simulink model "servo_sim"  (R2023a)
settings: configuration reference "config" (kept outside this file)
model workspace (MATLAB code in the model file + MAT data in the model file):
  cmdLim = Simulink.Parameter
  cmdLim.Value = 15
  cmdLim.Description = 'Limit for controlling the maximum surface command angle.'
  cmdLim.Min = 0
  cmdLim.Max = 90
  cmdLim.DocUnits = 'deg'
  dispGain = Simulink.Parameter
  dispGain.Value = 0.75
  dispGain.Description = 'Gain applied to the displacement error.'
  dispGain.Min = 0
  dispGain.Max = []
  dispGain.DocUnits = 'deg/sec/deg'
  dispLim = Simulink.Parameter
  dispLim.Value = 30
  dispLim.Description = 'Limit for controlling the maximum commanded angle.'
  dispLim.Min = 0
  dispLim.Max = 180
  dispLim.DocUnits = 'deg'
  intGain = Simulink.Parameter
  intGain.Value = 0.5
  intGain.Description = 'Gain applied to the integral error.'
  intGain.Min = 0
  intGain.Max = []
  intGain.DocUnits = 'deg/sec/deg/sec'
  intLim = Simulink.Parameter
  intLim.Value = 5
  intLim.Description = 'Limit for controlling the maximum commanded angle.'
  intLim.Min = 0
  intLim.Max = 90
  intLim.DocUnits = 'deg'
  rateGain = Simulink.Parameter
  rateGain.Value = 2
  rateGain.Description = 'Gain applied to the rate error.'
  rateGain.Min = 0
  rateGain.Max = []
  rateGain.DocUnits = 'deg/deg/sec'
  rateLim = Simulink.Parameter
  rateLim.Value = 6
  rateLim.Description = 'Limit for controlling the maximum commanded angle.'
  rateLim.Min = 0
  rateLim.Max = 180
  rateLim.DocUnits = 'deg/sec'
  hdgGain = Simulink.Parameter
  hdgGain.Value = 0.015
  b = Simulink.Parameter
  b.Value = 0.001
  b.DataType = 'single'
  b.Complexity = 'real'
  b.Dimensions = [1 1]
  enc_line = Simulink.Parameter
  enc_line.Value = 10000
  enc_line.DataType = 'single'
  enc_line.Complexity = 'real'
  enc_line.Dimensions = [1 1]
  fc = Simulink.Parameter
  fc.Value = 0.001
  fc.DataType = 'single'
  fc.Complexity = 'real'
  fc.Dimensions = [1 1]
  flux = Simulink.Parameter
  flux.Value = 0.0125
  flux.DataType = 'single'
  flux.Complexity = 'real'
  flux.Dimensions = [1 1]
  fs = Simulink.Parameter
  fs.Value = 10000
  fs.Description = '位置环 速度环执行频率'
  fs.DataType = 'single'
  fs.Complexity = 'real'
  fs.Dimensions = [1 1]
  j = Simulink.Parameter
  j.Value = 1.9e-05
  j.DataType = 'single'
  j.Complexity = 'real'
  j.Dimensions = [1 1]
  j_inv = Simulink.Parameter
  j_inv.Value = 52631.5789474
  j_inv.DataType = 'single'
  j_inv.Complexity = 'real'
  j_inv.Dimensions = [1 1]
  kt = Simulink.Parameter
  kt.Value = 0.075
  kt.DataType = 'single'
  kt.Complexity = 'real'
  kt.Dimensions = [1 1]
  ld = Simulink.Parameter
  ld.Value = 0.00085
  ld.DataType = 'single'
  ld.Complexity = 'real'
  ld.Dimensions = [1 1]
  ld_inv = Simulink.Parameter
  ld_inv.Value = 1176.47058824
  ld_inv.DataType = 'single'
  ld_inv.Complexity = 'real'
  ld_inv.Dimensions = [1 1]
  lq = Simulink.Parameter
  lq.Value = 0.00085
  lq.DataType = 'single'
  lq.Complexity = 'real'
  lq.Dimensions = [1 1]
  lq_inv = Simulink.Parameter
  lq_inv.Value = 1176.47058824
  lq_inv.DataType = 'single'
  lq_inv.Complexity = 'real'
  lq_inv.Dimensions = [1 1]
  pn = Simulink.Parameter
  pn.Value = 4
  pn.DataType = 'single'
  pn.Complexity = 'real'
  pn.Dimensions = [1 1]
  r = Simulink.Parameter
  r.Value = 0.649
  r.DataType = 'single'
  r.Complexity = 'real'
  r.Dimensions = [1 1]
  tc = Simulink.Parameter
  tc.Value = 5e-05
  tc.Description = '电流环运行频率用来设定综合仿真的参数'
  tc.DataType = 'double'
  tc.Complexity = 'real'
  tc.Dimensions = [1 1]
  tp = Simulink.Parameter
  tp.Value = 0.0001
  tp.Description = '位置环速度环执行周期'
  tp.DataType = 'double'
  tp.Complexity = 'real'
  tp.Dimensions = [1 1]
  ts = Simulink.Parameter
  ts.Value = 1e-05
  ts.Description = '模型仿真的周期 s'
  ts.DataType = 'double'
  ts.Complexity = 'real'
  ts.Dimensions = [1 1]
settings Model: RequirementInfo={} %GIDa_fe9045fd_0412_4b6e_8206_617cc20e6fde  DataDictionary=model_config.sldd  ParameterArgumentNames=b,enc_line,fc,flux,fs,j,j_inv,kt,ld,ld_inv,lq,lq_inv,pn,r  Creator=Administrator  LastModifiedBy=Administrator
settings ConfigSetRef: SourceName=config

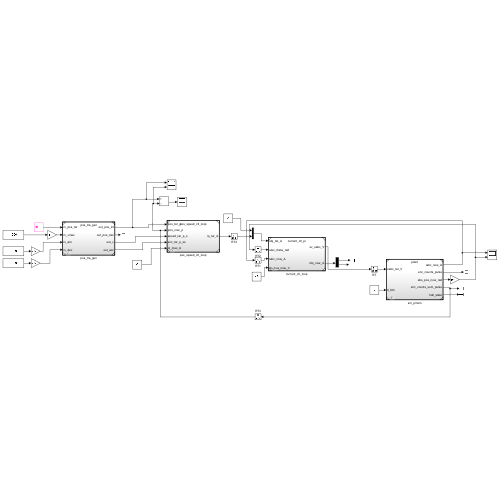
[thumbnail: Simulink's stored preview of the top-level diagram]
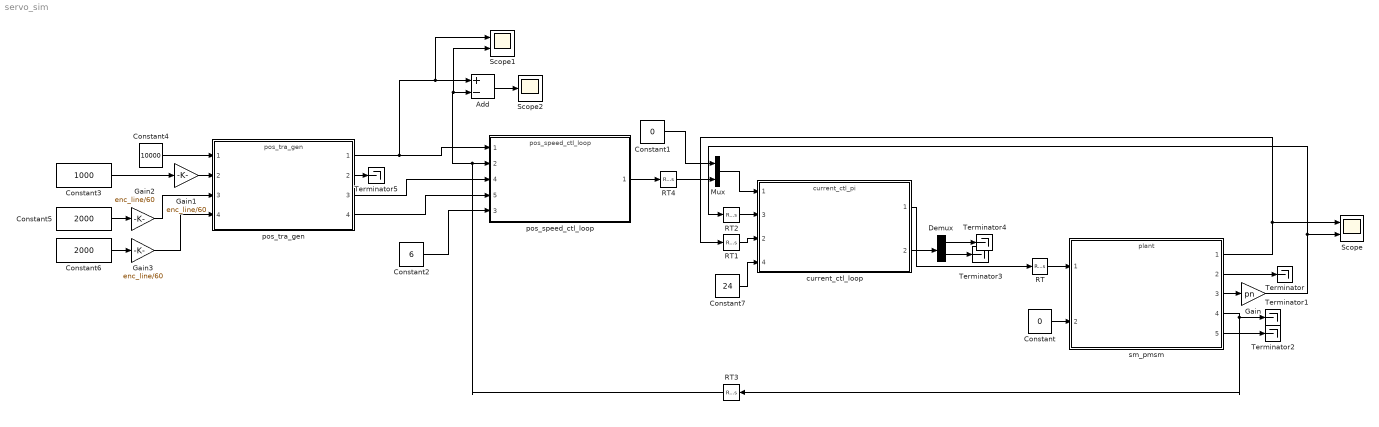
== system servo_sim ==
  Add : Sum  Inputs=+-
  Constant : Constant  Value=0  OutDataTypeStr=single
  Constant1 : Constant  Value=0  OutDataTypeStr=single
  Constant2 : Constant  Value=6  OutDataTypeStr=single
  Constant3 : Constant  Value=1000  OutDataTypeStr=single
  Constant4 : Constant  Value=10000  OutDataTypeStr=int64
  Constant5 : Constant  Value=2000  OutDataTypeStr=single
  Constant6 : Constant  Value=2000  OutDataTypeStr=single
  Constant7 : Constant  Value=24  OutDataTypeStr=single
  Demux : Demux  Outputs=2
  Gain : Gain  Gain=pn
  Gain1 : Gain  Gain=enc_line/60
  Gain2 : Gain  Gain=enc_line/60
  Gain3 : Gain  Gain=enc_line/60
  Mux : Mux  Inputs=2
  RT : RateTransition  OutPortSampleTime=ts
  RT1 : RateTransition  OutPortSampleTime=tc
  RT2 : RateTransition  OutPortSampleTime=tc
  RT3 : RateTransition  OutPortSampleTime=tp
  RT4 : RateTransition  OutPortSampleTime=tc
  Scope : Scope  NumInputPorts=2
  Scope1 : Scope  NumInputPorts=2
  Scope2 : Scope
  Terminator{,1..5} (6 alike) : Terminator
  current_ctl_loop : ModelReference  ModelNameDialog=current_ctl_pi.slx  UsingDefaultArgumentValue=0,0,0,0,0,0,0,0,0  SimulationMode=Normal  ModelReferenceVersion=2.138
      settings: PortSchema="{\"entries\":[{\"content\":{\"sides\":[{\"content\":{\"connectorIds\":[\"In1\",\"In3\",\"In2\",\"In4\"]},\"type\":\"ConnectorPlacement.EquallySpacedRectSide\",\"uuid\":\"465030fc-d4ed-4fad-a179-540c34c84031\"},{\"content\":{\"connectorIds\":[\"Out1\",\"Out2\"],\"side\":\"RIGHT\"},\"type\":\"ConnectorPlacement.EquallySpacedRectSide\",\"uuid\":\"fab44f7c-49ff-4c48-be02-a76080765122\"},{\"content\":{\"side\":\"TOP\"},\"type\":\"ConnectorPlacement.EquallySpacedRectSide\",\"uuid\":\"fa8fd0f2-cfd7-4f03-a40d-8124b2b913be\"}]},\"type\":\"ConnectorPlacement.EquallySpacedConnector\",\"uuid\":\"0e10ec8c-f9f2-4aaa-bb2e-fccf0700d204\"}],\"packageUris\":[\"http://schema.mathworks.com/mf0/Connector/R2020b\"],\"version\":\"1.0\"}"
  pos_speed_ctl_loop : ModelReference  ModelNameDialog=pos_speed_ctl_loop.slx  UsingDefaultArgumentValue=0,0,0,0,0,0,0,0,0,0,0,0,0,0,0,0,0  SimulationMode=Normal  ModelReferenceVersion=2.804
      settings: PortSchema="{\"entries\":[{\"content\":{\"sides\":[{\"content\":{\"connectorIds\":[\"In1\",\"In2\",\"In4\",\"In5\",\"In3\"]},\"type\":\"ConnectorPlacement.EquallySpacedRectSide\",\"uuid\":\"5ddb49bb-ac5d-4f8e-87f7-0b935d8e9e65\"},{\"content\":{\"connectorIds\":[\"Out1\"],\"side\":\"RIGHT\"},\"type\":\"ConnectorPlacement.EquallySpacedRectSide\",\"uuid\":\"c90d95c4-1bc5-43ed-9064-d0ad7fcbaa61\"},{\"content\":{\"side\":\"TOP\"},\"type\":\"ConnectorPlacement.EquallySpacedRectSide\",\"uuid\":\"9c3e5f13-9f26-4630-97bb-51641d37a8f2\"}]},\"type\":\"ConnectorPlacement.EquallySpacedConnector\",\"uuid\":\"bf3fc3ad-e940-4a2f-a6fe-e6447d4e0dfa\"}],\"packageUris\":[\"http://schema.mathworks.com/mf0/Connector/R2020b\"],\"version\":\"1.0\"}"
  pos_tra_gen : ModelReference  ModelNameDialog=pos_tra_gen.slx  UsingDefaultArgumentValue=0  SimulationMode=Normal  ModelReferenceVersion=2.26
  sm_pmsm : ModelReference  ModelNameDialog=plant.slx  UsingDefaultArgumentValue=0,0,0,0,0,0,0,0,0,0,0,0,0,0,0  SimulationMode=Normal  ModelReferenceVersion=1.22
  wires:
  Constant/1 -> sm_pmsm/2
  current_ctl_loop/1 -> RT/1
  Constant1/1 -> Mux/1
  Mux/1 -> current_ctl_loop/1
  sm_pmsm/3 -> Gain/1
  sm_pmsm/2 -> Terminator/1
  sm_pmsm/5 -> Terminator2/1
  RT/1 -> sm_pmsm/1
  sm_pmsm/1 -> Scope/1, RT1/1
  Gain/1 -> RT2/1, Scope/2
  current_ctl_loop/2 -> Demux/1
  RT2/1 -> current_ctl_loop/3
  Constant2/1 -> pos_speed_ctl_loop/3
  Add/1 -> Scope2/1
  pos_speed_ctl_loop/1 -> RT4/1
  sm_pmsm/4 -> Terminator1/1, RT3/1
  Demux/2 -> Terminator3/1
  RT1/1 -> current_ctl_loop/2
  Demux/1 -> Terminator4/1
  Constant4/1 -> pos_tra_gen/1
  Constant3/1 -> Gain1/1
  Constant5/1 -> Gain2/1
  Constant6/1 -> Gain3/1
  pos_tra_gen/1 -> Scope1/1, Add/1, pos_speed_ctl_loop/1
  pos_tra_gen/2 -> Terminator5/1
  pos_tra_gen/3 -> pos_speed_ctl_loop/4
  pos_tra_gen/4 -> pos_speed_ctl_loop/5
  RT3/1 -> pos_speed_ctl_loop/2, Scope1/2, Add/2
  RT4/1 -> Mux/2
  Gain1/1 -> pos_tra_gen/2
  Gain2/1 -> pos_tra_gen/3
  Gain3/1 -> pos_tra_gen/4
  Constant7/1 -> current_ctl_loop/4
